simulink model "slidingModeControl"  (R2018a)
settings: Solver=VariableStepAuto  StartTime=0.0  StopTime=100  RelTol=1e-3
settings Model: Creator=Haydar  LastModifiedBy=Haydar
settings SolverCC: MaxConsecutiveZCs=10000

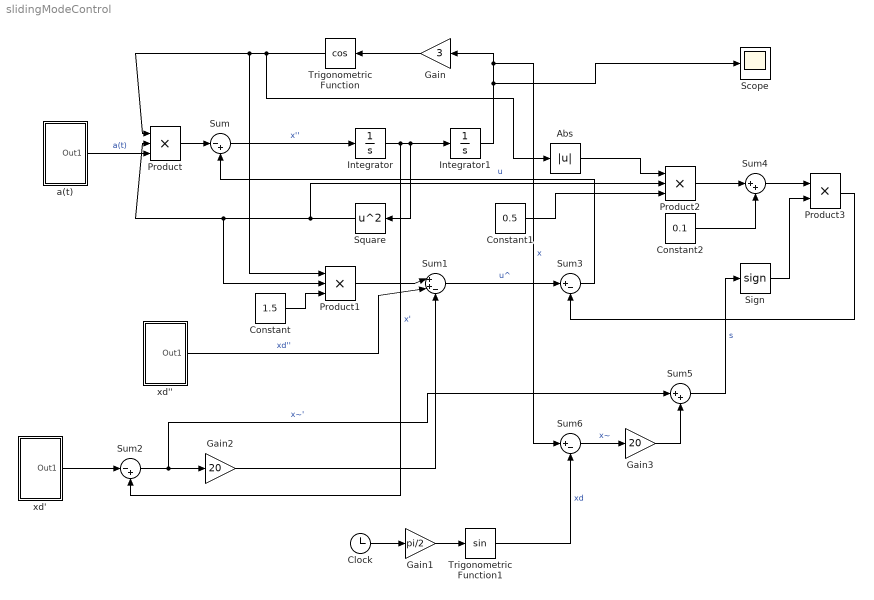
== system slidingModeControl ==
  Abs : Abs
  Clock : Clock
  Constant : Constant  Value=1.5
  Constant1 : Constant  Value=0.5
  Constant2 : Constant  Value=0.1
  Gain : Gain  Gain=3
  Gain1 : Gain  Gain=pi/2
  Gain2 : Gain  Gain=20
  Gain3 : Gain  Gain=20
  Integrator : Integrator
  Integrator1 : Integrator
  Product : Product  Inputs=3
  Product1 : Product  Inputs=3
  Product2 : Product  Inputs=3
  Product3 : Product
  Scope : Scope
  Sign : Signum
  Square : Math  Operator=square  SaturateOnIntegerOverflow=on
  Sum : Sum  Inputs=|-+
  Sum1 : Sum  Inputs=|++-
  Sum2 : Sum  Inputs=|-+
  Sum3 : Sum  Inputs=|+-
  Sum4 : Sum  Inputs=|++
  Sum5 : Sum  Inputs=|++
  Sum6 : Sum  Inputs=|+-
  Trigonometric Function : Trigonometry  Operator=cos
  Trigonometric Function1 : Trigonometry
  "a(t) " : Subsystem
  xd' : Subsystem
  xd'' : Subsystem
  wires:
  Sum/1 -> Integrator/1  "x''"
  Integrator/1 -> Integrator1/1, Square/1, Sum2/2  "x'"
  Square/1 -> Product2/2, Product1/2, Product/2
  Integrator1/1 -> Scope/1, Sum6/1, Gain/1  "x"
  Gain/1 -> Trigonometric Function/1
  Product/1 -> Sum/1
  Trigonometric Function/1 -> Abs/1, Product/1, Product1/1
  "a(t) "/1(Out1) -> Product/3  "a(t)"
  Constant/1 -> Product1/3
  Clock/1 -> Gain1/1
  Gain1/1 -> Trigonometric Function1/1
  Trigonometric Function1/1 -> Sum6/2  "xd"
  Product1/1 -> Sum1/1
  Sum2/1 -> Sum5/1, Gain2/1  "x~'"
  Gain2/1 -> Sum1/3
  Sum1/1 -> Sum3/1  "u^"
  Constant1/1 -> Product2/3
  Abs/1 -> Product2/1
  Constant2/1 -> Sum4/2
  Product2/1 -> Sum4/1
  Sum4/1 -> Product3/1
  Sign/1 -> Product3/2
  Sum6/1 -> Gain3/1  "x~"
  Gain3/1 -> Sum5/2
  Sum5/1 -> Sign/1  "s"
  Product3/1 -> Sum3/2
  Sum3/1 -> Sum/2  "u"
  xd'/1(Out1) -> Sum2/1
  xd''/1(Out1) -> Sum1/2  "xd''"

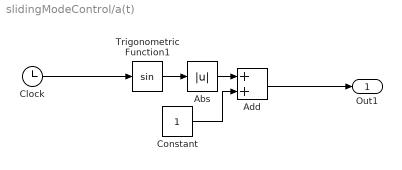
== system slidingModeControl/a(t)  ==
  Abs : Abs
  Add : Sum
  Clock : Clock
  Constant : Constant
  Trigonometric Function1 : Trigonometry
  Out1 : Outport
  wires:
  Clock/1 -> Trigonometric Function1/1
  Abs/1 -> Add/1
  Trigonometric Function1/1 -> Abs/1
  Add/1 -> Out1/1
  Constant/1 -> Add/2

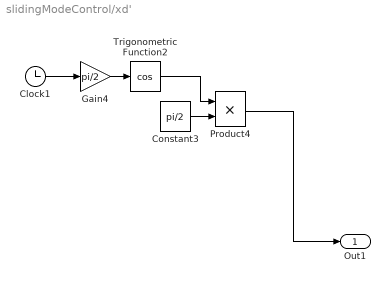
== system slidingModeControl/xd' ==
  Clock1 : Clock
  Constant3 : Constant  Value=pi/2
  Gain4 : Gain  Gain=pi/2
  Product4 : Product
  Trigonometric Function2 : Trigonometry  Operator=cos
  Out1 : Outport
  wires:
  Gain4/1 -> Trigonometric Function2/1
  Clock1/1 -> Gain4/1
  Constant3/1 -> Product4/2
  Trigonometric Function2/1 -> Product4/1
  Product4/1 -> Out1/1

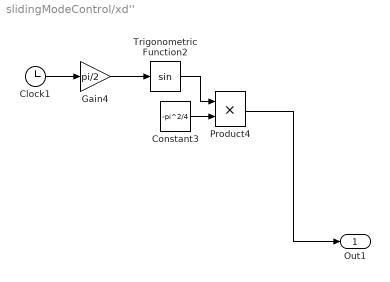
== system slidingModeControl/xd'' ==
  Clock1 : Clock
  Constant3 : Constant  Value=-pi^2/4
  Gain4 : Gain  Gain=pi/2
  Product4 : Product
  Trigonometric Function2 : Trigonometry
  Out1 : Outport
  wires:
  Product4/1 -> Out1/1
  Trigonometric Function2/1 -> Product4/1
  Constant3/1 -> Product4/2
  Clock1/1 -> Gain4/1
  Gain4/1 -> Trigonometric Function2/1
